simulink model "PID_controller"  (R2017a)
settings: Solver=VariableStepAuto  StartTime=0.0  StopTime=50  RelTol=1e-3
values from neighbouring files (symbols this model uses):
  Cs1 = tf(Kc1, [ti1 0])    [PID_controller_params.m]
  Cs2 = tf(Kc2, [ti2 0])    [PID_controller_params.m]
  Ds1 = tf([(Kc1*tf1)+(Kc1*td1) 1], [tf1 1])    [PID_controller_params.m]
  Ds2 = tf([(Kc2*tf2)+(Kc2*td2) 1], [tf2 1])    [PID_controller_params.m]
  Gs = tf([-1 0.4],[1 0.5 0.04])    [PID_controller_params.m]    (also in PI_controller_params.m = tf([0.1],[10 1]))
settings Model: Creator=adityaaaap  LastModifiedBy=adityaaaap

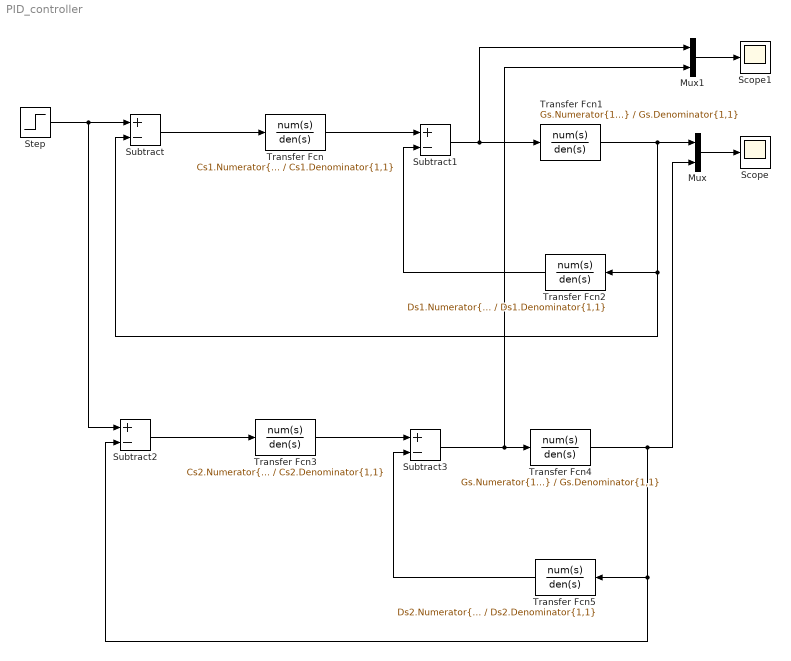
== system PID_controller ==
  Mux : Mux  Inputs=2
  Mux1 : Mux  Inputs=2
  Scope : Scope
  Scope1 : Scope
  Step : Step  Time=0  After=0.8  SampleTime=0
  Subtract{,1..3} (4 alike) : Sum  Inputs=+-
  Transfer Fcn : TransferFcn  Numerator=Cs1.Numerator{1,1}  Denominator=Cs1.Denominator{1,1}
  Transfer Fcn1 : TransferFcn  Numerator=Gs.Numerator{1,1}  Denominator=Gs.Denominator{1,1}
  Transfer Fcn2 : TransferFcn  Numerator=Ds1.Numerator{1,1}  Denominator=Ds1.Denominator{1,1}
  Transfer Fcn3 : TransferFcn  Numerator=Cs2.Numerator{1,1}  Denominator=Cs2.Denominator{1,1}
  Transfer Fcn4 : TransferFcn  Numerator=Gs.Numerator{1,1}  Denominator=Gs.Denominator{1,1}
  Transfer Fcn5 : TransferFcn  Numerator=Ds2.Numerator{1,1}  Denominator=Ds2.Denominator{1,1}
  wires:
  Step/1 -> Subtract2/1, Subtract/1
  Subtract/1 -> Transfer Fcn/1
  Transfer Fcn/1 -> Subtract1/1
  Subtract1/1 -> Mux1/1, Transfer Fcn1/1
  Transfer Fcn1/1 -> Transfer Fcn2/1, Subtract/2, Mux/1
  Mux/1 -> Scope/1
  Mux1/1 -> Scope1/1
  Transfer Fcn2/1 -> Subtract1/2
  Transfer Fcn4/1 -> Mux/2, Transfer Fcn5/1, Subtract2/2
  Transfer Fcn5/1 -> Subtract3/2
  Subtract3/1 -> Mux1/2, Transfer Fcn4/1
  Subtract2/1 -> Transfer Fcn3/1
  Transfer Fcn3/1 -> Subtract3/1
